simulink model "ME_423_Lab_1"  (R2024b)
settings: Solver=ode4  StartTime=0.0  StopTime=2600  FixedStep=1/1000  RelTol=1e-3
libraries: simulink x4
settings Model: Creator=fifty  LastModifiedBy=fifty

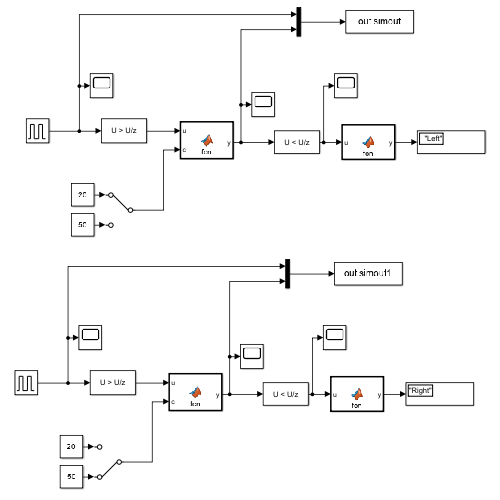
[thumbnail: Simulink's stored preview of the top-level diagram]
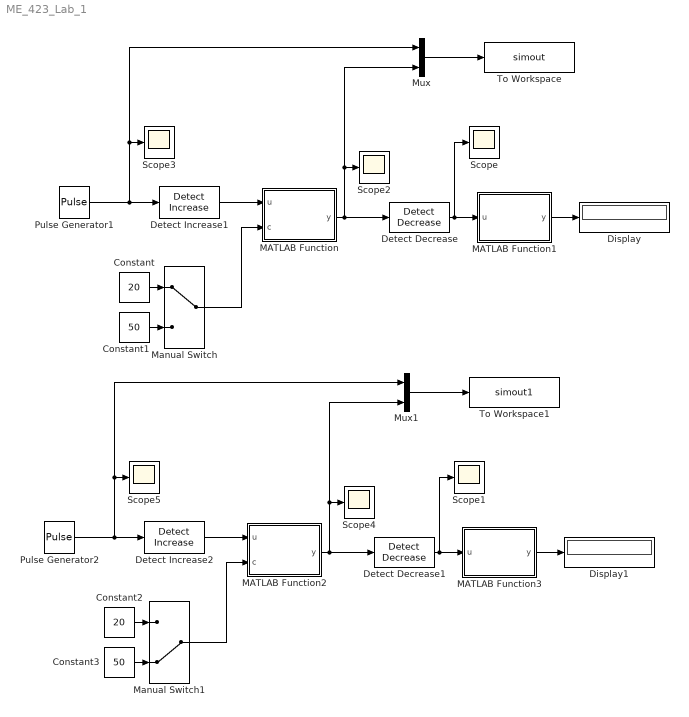
== system ME_423_Lab_1 ==
  Constant : Constant  Value=20
  Constant1 : Constant  Value=50
  Constant2 : Constant  Value=20
  Constant3 : Constant  Value=50
  Detect Decrease : simulink/Logic and Bit Operations/Detect Decrease  vinit=0.0  OutDataTypeStr=boolean
  Detect Decrease1 : simulink/Logic and Bit Operations/Detect Decrease  vinit=0.0  OutDataTypeStr=boolean
  Detect Increase1 : simulink/Logic and Bit Operations/Detect Increase  vinit=0.0  OutDataTypeStr=uint8
  Detect Increase2 : simulink/Logic and Bit Operations/Detect Increase  vinit=0.0  OutDataTypeStr=uint8
  Display : Display
  Display1 : Display
  MATLAB Function : MATLAB Function  TreatAsAtomicUnit=on
  MATLAB Function1 : MATLAB Function  TreatAsAtomicUnit=on
  MATLAB Function2 : MATLAB Function  TreatAsAtomicUnit=on
  MATLAB Function3 : MATLAB Function  TreatAsAtomicUnit=on
  Manual Switch : ManualSwitch
  Manual Switch1 : ManualSwitch  CurrentSetting=0
  Mux : Mux  Inputs=2
  Mux1 : Mux  Inputs=2
  Pulse Generator1 : DiscretePulseGenerator  PulseType=Time based  Amplitude=5  Period=10  PulseWidth=10
  Pulse Generator2 : DiscretePulseGenerator  PulseType=Time based  Amplitude=5  Period=10  PulseWidth=10
  Scope{,1..5} (6 alike) : Scope
  To Workspace : ToWorkspace  VariableName=simout  SampleTime=-1
  To Workspace1 : ToWorkspace  VariableName=simout1  SampleTime=-1
  wires:
  Pulse Generator1/1 -> Scope3/1, Mux/1, Detect Increase1/1
  Detect Increase1/1 -> MATLAB Function/1(u)
  MATLAB Function/1(y) -> Detect Decrease/1, Mux/2, Scope2/1
  Constant/1 -> Manual Switch/1
  Constant1/1 -> Manual Switch/2
  Manual Switch/1 -> MATLAB Function/2(c)
  Detect Decrease/1 -> Scope/1, MATLAB Function1/1(u)
  MATLAB Function1/1(y) -> Display/1
  Mux/1 -> To Workspace/1
  Mux1/1 -> To Workspace1/1
  MATLAB Function3/1(y) -> Display1/1
  Constant3/1 -> Manual Switch1/2
  Manual Switch1/1 -> MATLAB Function2/2(c)
  Constant2/1 -> Manual Switch1/1
  Pulse Generator2/1 -> Scope5/1, Mux1/1, Detect Increase2/1
  MATLAB Function2/1(y) -> Detect Decrease1/1, Mux1/2, Scope4/1
  Detect Increase2/1 -> MATLAB Function2/1(u)
  Detect Decrease1/1 -> Scope1/1, MATLAB Function3/1(u)

== matlab function ME_423_Lab_1/MATLAB Function ==
  data: u input; y output; c input
function y = fcn(u, c)

persistent x;

if isempty(x)
    x = 0;
end

if u == 1
    x = x + 1;
    if x == c+1
        x = 0;
    end
end
y = x;

== matlab function ME_423_Lab_1/MATLAB Function2 ==
  data: u input; y output; c input
function y = fcn(u, c)

persistent x;

if isempty(x)
    x = 0;
end

if u == 1
    x = x + 1;
    if x == c+1
        x = 0;
    end
end
y = x;

== matlab function ME_423_Lab_1/MATLAB Function3 ==
  data: u input; y output
function y = fcn(u)

persistent x

if isempty(x)
    x = 0;
end

if u == 1
    x = x +1;
end

u = x;

if mod(u,2) == 0
    y = "Left";
else 
    y = "Right";
end

== matlab function ME_423_Lab_1/MATLAB Function1 ==
  data: u input; y output
function y = fcn(u)

persistent x

if isempty(x)
    x = 0;
end

if u == 1
    x = x +1;
end

u = x;

if mod(u,2) == 0
    y = "Left";
else 
    y = "Right";
end
